simulink model "dcmg"  (R2020a)
settings: Solver=VariableStepAuto  StartTime=0.0  StopTime=Inf  FixedStep=50e-6  RelTol=1e-3
PostLoadFcn:
  | , if any(exist('dsrtsu_mdlpostloadfcn', 'file') ~= 0), dsrtsu_mdlpostloadfcn('Execute', bdroot); end,
InitFcn:
  | , if any(exist('rtifpga_mdlclblib', 'file') ~= 0), rtifpga_mdlclblib('Init', bdroot); end,
model workspace (MAT data in the model file):
  FPGA_dcmg_1_Register_1_1_1_write : Simulink.Signal (value not decoded)
  FPGA_dcmg_1_Register_2_1_1_write : Simulink.Signal (value not decoded)
  FPGA_dcmg_1_Register_3_1_1_write : Simulink.Signal (value not decoded)
  FPGA_dcmg_1_Register_4_1_1_write : Simulink.Signal (value not decoded)
  FPGA_dcmg_1_Register_5_1_1_write : Simulink.Signal (value not decoded)
values from neighbouring files (symbols this model uses):
  den = [1, zeros(1,499)]    [params.m]
  fixedgain_i = 10*1000/(3*100)    (= 33.3333333333)    [param.m]    (also in params.m)
  fixedgain_ibat = 10*1000/(3*100)    (= 33.3333333333)    [params.m]
  fixedgain_ipv = 10*1000/(3*100)    (= 33.3333333333)    [params.m]
  fixedgain_v = 10*22000/(3*100*2.5)    (= 293.333333333)    [params.m]
  fixedgain_vdc = 10*22000/(3*100*2.5)    (= 293.333333333)    [param.m]    (also in params.m = 586.666666667)
  fixedgain_vpv = 10*10000/(3*100*2.5)    (= 133.333333333)    [params.m]
  gain_iavsi = 1    [params.m]
  gain_ibat = 1    [params.m]
  gain_ibvsi = 1    [params.m]
  gain_icvsi = 1    [params.m]
  gain_ioavsi = 1    [params.m]
  gain_iobvsi = 1    [params.m]
  gain_ipv = 1    [params.m]
  gain_sinwave = 0.3    [params.m]
  gain_vavsi = 1    [params.m]
  gain_vbvsi = 1    [params.m]
  gain_vcvsi = 1    [params.m]
  gain_vdc = 1    [param.m]    (also in params.m)
  gain_vpv = 1    [params.m]
  N = 10    [param.m]    (also in params.m = 100)
  num = 1/500*ones(1,500)    [params.m]
  offset_iavsi = 0.2    [params.m]
  offset_ibat = 0    [params.m]
  offset_ibvsi = 0.2    [params.m]
  offset_icvsi = 0.2    [params.m]
  offset_ioavsi = 0    [params.m]
  offset_iobvsi = 0    [params.m]
  offset_ipv = 0    [params.m]
  offset_vavsi = 0    [params.m]
  offset_vbvsi = 0    [params.m]
  offset_vcvsi = 0    [params.m]
  offset_vdc = 1.5    [param.m]    (also in params.m = 0)
  offset_vpv = 0    [params.m]
  v_dc_ref = 40    [param.m]    (also in params.m = 24)
libraries: xbsIndex_r4 x258, rti1202lib_adc_class1 x10, rtiproclib x9, simulink x5, rti1202lib_adc_class2 x2, rtifpgainterfacelib x1
(part 7 of 7)

== system dcmg/fpga_dcmg/FPGA_XDATA_READ_BL1/phs_read_register/phs//rtlib_sim_model ==
  note: - The double to fixed-point conversion done by the XSG gateway behaves differently
      | than the conversion done by the RTLib C-code. Therefore the C-Code behaviour
      | is simulated via an s-function using the RTLib conversion technique including scaling and saturation.
  data_i1 : Inport
  S-Function : S-Function  FunctionName=DS1302_read_register  Parameters=mode;binaryPoint  SFunctionDeploymentMode=off  EnableBusSupport=off
  Zero-Order Hold : ZeroOrderHold  SampleTime=proc_sample_time
  data_o1 : Outport  VectorParamsAs1DForOutWhenUnconnected=off
  wires:
  Zero-Order Hold/1 -> S-Function/1
  S-Function/1 -> data_o1/1
  data_i1/1 -> Zero-Order Hold/1

== system dcmg/fpga_dcmg/FPGA_XDATA_READ_BL2/phs_read_register/com_fct_model ==
  note: - Register data is presented to the FPGA application without data adaptions.
      |
      | - Register group accesses are implicitly simulated by simulink: all FPGA
      | communication function interface blocks are simulated within one task
      | with a unique sample time --> in- and ouputs are sampled simultaneously
      | and therefore data consistency is guaranteed.
  data_i1 : Inport
  Data_New_Calc : Subsystem
  Zero-Order Hold : ZeroOrderHold  SampleTime=fpga_sample_time
  data_o1 : Outport  VectorParamsAs1DForOutWhenUnconnected=off
  data_new_o : Outport  Port=2  VectorParamsAs1DForOutWhenUnconnected=off
  wires:
  Zero-Order Hold/1 -> data_o1/1
  Data_New_Calc/1(Out1) -> data_new_o/1
  data_i1/1 -> Zero-Order Hold/1, Data_New_Calc/1(In1)

== system dcmg/fpga_dcmg/FPGA_XDATA_READ_BL2/phs_read_register/phs//rtlib_sim_model ==
  note: - The double to fixed-point conversion done by the XSG gateway behaves differently
      | than the conversion done by the RTLib C-code. Therefore the C-Code behaviour
      | is simulated via an s-function using the RTLib conversion technique including scaling and saturation.
  data_i1 : Inport
  S-Function : S-Function  FunctionName=DS1302_read_register  Parameters=mode;binaryPoint  SFunctionDeploymentMode=off  EnableBusSupport=off
  Zero-Order Hold : ZeroOrderHold  SampleTime=proc_sample_time
  data_o1 : Outport  VectorParamsAs1DForOutWhenUnconnected=off
  wires:
  Zero-Order Hold/1 -> S-Function/1
  S-Function/1 -> data_o1/1
  data_i1/1 -> Zero-Order Hold/1

== system dcmg/fpga_dcmg/FPGA_XDATA_READ_BL3/phs_read_register/com_fct_model ==
  note: - Register data is presented to the FPGA application without data adaptions.
      |
      | - Register group accesses are implicitly simulated by simulink: all FPGA
      | communication function interface blocks are simulated within one task
      | with a unique sample time --> in- and ouputs are sampled simultaneously
      | and therefore data consistency is guaranteed.
  data_i1 : Inport
  Data_New_Calc : Subsystem
  Zero-Order Hold : ZeroOrderHold  SampleTime=fpga_sample_time
  data_o1 : Outport  VectorParamsAs1DForOutWhenUnconnected=off
  data_new_o : Outport  Port=2  VectorParamsAs1DForOutWhenUnconnected=off
  wires:
  Zero-Order Hold/1 -> data_o1/1
  Data_New_Calc/1(Out1) -> data_new_o/1
  data_i1/1 -> Zero-Order Hold/1, Data_New_Calc/1(In1)

== system dcmg/fpga_dcmg/FPGA_XDATA_READ_BL3/phs_read_register/phs//rtlib_sim_model ==
  note: - The double to fixed-point conversion done by the XSG gateway behaves differently
      | than the conversion done by the RTLib C-code. Therefore the C-Code behaviour
      | is simulated via an s-function using the RTLib conversion technique including scaling and saturation.
  data_i1 : Inport
  S-Function : S-Function  FunctionName=DS1302_read_register  Parameters=mode;binaryPoint  SFunctionDeploymentMode=off  EnableBusSupport=off
  Zero-Order Hold : ZeroOrderHold  SampleTime=proc_sample_time
  data_o1 : Outport  VectorParamsAs1DForOutWhenUnconnected=off
  wires:
  Zero-Order Hold/1 -> S-Function/1
  S-Function/1 -> data_o1/1
  data_i1/1 -> Zero-Order Hold/1

== system dcmg/fpga_dcmg/FPGA_XDATA_READ_BL4/phs_read_register/com_fct_model ==
  note: - Register data is presented to the FPGA application without data adaptions.
      |
      | - Register group accesses are implicitly simulated by simulink: all FPGA
      | communication function interface blocks are simulated within one task
      | with a unique sample time --> in- and ouputs are sampled simultaneously
      | and therefore data consistency is guaranteed.
  data_i1 : Inport
  Data_New_Calc : Subsystem
  Zero-Order Hold : ZeroOrderHold  SampleTime=fpga_sample_time
  data_o1 : Outport  VectorParamsAs1DForOutWhenUnconnected=off
  data_new_o : Outport  Port=2  VectorParamsAs1DForOutWhenUnconnected=off
  wires:
  Zero-Order Hold/1 -> data_o1/1
  Data_New_Calc/1(Out1) -> data_new_o/1
  data_i1/1 -> Zero-Order Hold/1, Data_New_Calc/1(In1)

== system dcmg/fpga_dcmg/FPGA_XDATA_READ_BL4/phs_read_register/phs//rtlib_sim_model ==
  note: - The double to fixed-point conversion done by the XSG gateway behaves differently
      | than the conversion done by the RTLib C-code. Therefore the C-Code behaviour
      | is simulated via an s-function using the RTLib conversion technique including scaling and saturation.
  data_i1 : Inport
  S-Function : S-Function  FunctionName=DS1302_read_register  Parameters=mode;binaryPoint  SFunctionDeploymentMode=off  EnableBusSupport=off
  Zero-Order Hold : ZeroOrderHold  SampleTime=proc_sample_time
  data_o1 : Outport  VectorParamsAs1DForOutWhenUnconnected=off
  wires:
  Zero-Order Hold/1 -> S-Function/1
  S-Function/1 -> data_o1/1
  data_i1/1 -> Zero-Order Hold/1

== system dcmg/fpga_dcmg/FPGA_XDATA_READ_BL5/phs_read_register/com_fct_model ==
  note: - Register data is presented to the FPGA application without data adaptions.
      |
      | - Register group accesses are implicitly simulated by simulink: all FPGA
      | communication function interface blocks are simulated within one task
      | with a unique sample time --> in- and ouputs are sampled simultaneously
      | and therefore data consistency is guaranteed.
  data_i1 : Inport
  Data_New_Calc : Subsystem
  Zero-Order Hold : ZeroOrderHold  SampleTime=fpga_sample_time
  data_o1 : Outport  VectorParamsAs1DForOutWhenUnconnected=off
  data_new_o : Outport  Port=2  VectorParamsAs1DForOutWhenUnconnected=off
  wires:
  Zero-Order Hold/1 -> data_o1/1
  Data_New_Calc/1(Out1) -> data_new_o/1
  data_i1/1 -> Zero-Order Hold/1, Data_New_Calc/1(In1)

== system dcmg/fpga_dcmg/FPGA_XDATA_READ_BL5/phs_read_register/phs//rtlib_sim_model ==
  note: - The double to fixed-point conversion done by the XSG gateway behaves differently
      | than the conversion done by the RTLib C-code. Therefore the C-Code behaviour
      | is simulated via an s-function using the RTLib conversion technique including scaling and saturation.
  data_i1 : Inport
  S-Function : S-Function  FunctionName=DS1302_read_register  Parameters=mode;binaryPoint  SFunctionDeploymentMode=off  EnableBusSupport=off
  Zero-Order Hold : ZeroOrderHold  SampleTime=proc_sample_time
  data_o1 : Outport  VectorParamsAs1DForOutWhenUnconnected=off
  wires:
  Zero-Order Hold/1 -> S-Function/1
  S-Function/1 -> data_o1/1
  data_i1/1 -> Zero-Order Hold/1

== system dcmg/RTI Data/RTI Data Store/RTI Data Store/RTI Data Store/RTI Data Store ==

== system dcmg/fpga_dcmg/FPGA_INT_BL1/phs_interrupt/phs//rtlib_sim_model/Triggered Subsystem ==
  Trigger : TriggerPort  VariantControl=(inherit)
  Function-Call Generator : simulink/Ports & Subsystems/Function-Call Generator  sample_time=-1  numberOfIterations=1
  Out1 : Outport  VectorParamsAs1DForOutWhenUnconnected=off
  wires:
  Function-Call Generator/1 -> Out1/1

== system dcmg/fpga_dcmg/FPGA_INT_BL2/phs_interrupt/phs//rtlib_sim_model/Triggered Subsystem ==
  Trigger : TriggerPort  VariantControl=(inherit)
  Function-Call Generator : simulink/Ports & Subsystems/Function-Call Generator  sample_time=-1  numberOfIterations=1
  Out1 : Outport  VectorParamsAs1DForOutWhenUnconnected=off
  wires:
  Function-Call Generator/1 -> Out1/1

== system dcmg/fpga_dcmg/FPGA_INT_BL3/phs_interrupt/phs//rtlib_sim_model/Triggered Subsystem ==
  Trigger : TriggerPort  VariantControl=(inherit)
  Function-Call Generator : simulink/Ports & Subsystems/Function-Call Generator  sample_time=-1  numberOfIterations=1
  Out1 : Outport  VectorParamsAs1DForOutWhenUnconnected=off
  wires:
  Function-Call Generator/1 -> Out1/1

== system dcmg/fpga_dcmg/FPGA_XDATA_READ_BL1/phs_read_register/com_fct_model/Data_New_Calc ==
  note: The new data flag is presented whenever the input data port is sampled.
      | The flag is set to 1 for one FPGA simulation step and reset to 0 for the
      | remaining FPGA simulation steps contained within one processor simulation step.
  In1 : Inport
  Add : Sum
  Constant : Constant  Value=fpga_sample_time  SampleTime=fpga_sample_time
  Constant1 : Constant  Value=0
  Divide : Product  Inputs=*/
  Divide1 : Product  Inputs=*/
  Math Function : Math  Operator=mod  SignedPower=on  SaturateOnIntegerOverflow=on
  Relational Operator : RelationalOperator  Operator===  OutDataTypeStr=boolean  RndMeth=Nearest
  Unit Delay1 : UnitDelay  InitialCondition=-1  SampleTime=-1  HasFrameUpgradeWarning=on
  Weighted Sample Time1 : SampleTimeMath  TsampMathOp=Ts Only
  Out1 : Outport  VectorParamsAs1DForOutWhenUnconnected=off
  wires:
  Constant/1 -> Divide1/2, Divide1/1, Divide/2
  Weighted Sample Time1/1 -> Divide/1
  Math Function/1 -> Relational Operator/1
  Relational Operator/1 -> Out1/1
  In1/1 -> Weighted Sample Time1/1
  Divide1/1 -> Add/1
  Unit Delay1/1 -> Add/2
  Add/1 -> Unit Delay1/1, Math Function/1
  Constant1/1 -> Relational Operator/2
  Divide/1 -> Math Function/2

== system dcmg/fpga_dcmg/FPGA_XDATA_READ_BL2/phs_read_register/com_fct_model/Data_New_Calc ==
  note: The new data flag is presented whenever the input data port is sampled.
      | The flag is set to 1 for one FPGA simulation step and reset to 0 for the
      | remaining FPGA simulation steps contained within one processor simulation step.
  In1 : Inport
  Add : Sum
  Constant : Constant  Value=fpga_sample_time  SampleTime=fpga_sample_time
  Constant1 : Constant  Value=0
  Divide : Product  Inputs=*/
  Divide1 : Product  Inputs=*/
  Math Function : Math  Operator=mod  SignedPower=on  SaturateOnIntegerOverflow=on
  Relational Operator : RelationalOperator  Operator===  OutDataTypeStr=boolean  RndMeth=Nearest
  Unit Delay1 : UnitDelay  InitialCondition=-1  SampleTime=-1  HasFrameUpgradeWarning=on
  Weighted Sample Time1 : SampleTimeMath  TsampMathOp=Ts Only
  Out1 : Outport  VectorParamsAs1DForOutWhenUnconnected=off
  wires:
  Constant/1 -> Divide1/2, Divide1/1, Divide/2
  Weighted Sample Time1/1 -> Divide/1
  Math Function/1 -> Relational Operator/1
  Relational Operator/1 -> Out1/1
  In1/1 -> Weighted Sample Time1/1
  Divide1/1 -> Add/1
  Unit Delay1/1 -> Add/2
  Add/1 -> Unit Delay1/1, Math Function/1
  Constant1/1 -> Relational Operator/2
  Divide/1 -> Math Function/2

== system dcmg/fpga_dcmg/FPGA_XDATA_READ_BL3/phs_read_register/com_fct_model/Data_New_Calc ==
  note: The new data flag is presented whenever the input data port is sampled.
      | The flag is set to 1 for one FPGA simulation step and reset to 0 for the
      | remaining FPGA simulation steps contained within one processor simulation step.
  In1 : Inport
  Add : Sum
  Constant : Constant  Value=fpga_sample_time  SampleTime=fpga_sample_time
  Constant1 : Constant  Value=0
  Divide : Product  Inputs=*/
  Divide1 : Product  Inputs=*/
  Math Function : Math  Operator=mod  SignedPower=on  SaturateOnIntegerOverflow=on
  Relational Operator : RelationalOperator  Operator===  OutDataTypeStr=boolean  RndMeth=Nearest
  Unit Delay1 : UnitDelay  InitialCondition=-1  SampleTime=-1  HasFrameUpgradeWarning=on
  Weighted Sample Time1 : SampleTimeMath  TsampMathOp=Ts Only
  Out1 : Outport  VectorParamsAs1DForOutWhenUnconnected=off
  wires:
  Constant/1 -> Divide1/2, Divide1/1, Divide/2
  Weighted Sample Time1/1 -> Divide/1
  Math Function/1 -> Relational Operator/1
  Relational Operator/1 -> Out1/1
  In1/1 -> Weighted Sample Time1/1
  Divide1/1 -> Add/1
  Unit Delay1/1 -> Add/2
  Add/1 -> Unit Delay1/1, Math Function/1
  Constant1/1 -> Relational Operator/2
  Divide/1 -> Math Function/2

== system dcmg/fpga_dcmg/FPGA_XDATA_READ_BL4/phs_read_register/com_fct_model/Data_New_Calc ==
  note: The new data flag is presented whenever the input data port is sampled.
      | The flag is set to 1 for one FPGA simulation step and reset to 0 for the
      | remaining FPGA simulation steps contained within one processor simulation step.
  In1 : Inport
  Add : Sum
  Constant : Constant  Value=fpga_sample_time  SampleTime=fpga_sample_time
  Constant1 : Constant  Value=0
  Divide : Product  Inputs=*/
  Divide1 : Product  Inputs=*/
  Math Function : Math  Operator=mod  SignedPower=on  SaturateOnIntegerOverflow=on
  Relational Operator : RelationalOperator  Operator===  OutDataTypeStr=boolean  RndMeth=Nearest
  Unit Delay1 : UnitDelay  InitialCondition=-1  SampleTime=-1  HasFrameUpgradeWarning=on
  Weighted Sample Time1 : SampleTimeMath  TsampMathOp=Ts Only
  Out1 : Outport  VectorParamsAs1DForOutWhenUnconnected=off
  wires:
  Constant/1 -> Divide1/2, Divide1/1, Divide/2
  Weighted Sample Time1/1 -> Divide/1
  Math Function/1 -> Relational Operator/1
  Relational Operator/1 -> Out1/1
  In1/1 -> Weighted Sample Time1/1
  Divide1/1 -> Add/1
  Unit Delay1/1 -> Add/2
  Add/1 -> Unit Delay1/1, Math Function/1
  Constant1/1 -> Relational Operator/2
  Divide/1 -> Math Function/2

== system dcmg/fpga_dcmg/FPGA_XDATA_READ_BL5/phs_read_register/com_fct_model/Data_New_Calc ==
  note: The new data flag is presented whenever the input data port is sampled.
      | The flag is set to 1 for one FPGA simulation step and reset to 0 for the
      | remaining FPGA simulation steps contained within one processor simulation step.
  In1 : Inport
  Add : Sum
  Constant : Constant  Value=fpga_sample_time  SampleTime=fpga_sample_time
  Constant1 : Constant  Value=0
  Divide : Product  Inputs=*/
  Divide1 : Product  Inputs=*/
  Math Function : Math  Operator=mod  SignedPower=on  SaturateOnIntegerOverflow=on
  Relational Operator : RelationalOperator  Operator===  OutDataTypeStr=boolean  RndMeth=Nearest
  Unit Delay1 : UnitDelay  InitialCondition=-1  SampleTime=-1  HasFrameUpgradeWarning=on
  Weighted Sample Time1 : SampleTimeMath  TsampMathOp=Ts Only
  Out1 : Outport  VectorParamsAs1DForOutWhenUnconnected=off
  wires:
  Constant/1 -> Divide1/2, Divide1/1, Divide/2
  Weighted Sample Time1/1 -> Divide/1
  Math Function/1 -> Relational Operator/1
  Relational Operator/1 -> Out1/1
  In1/1 -> Weighted Sample Time1/1
  Divide1/1 -> Add/1
  Unit Delay1/1 -> Add/2
  Add/1 -> Unit Delay1/1, Math Function/1
  Constant1/1 -> Relational Operator/2
  Divide/1 -> Math Function/2

== matlab function dcmg/MPPT_system/MATLAB Function ==
  data: v_pv input; v_PandO output; i input; v_dc input; d output; P output
function [v_PandO, d, P] = MPPT(v_pv,i, v_dc)
persistent P_ant v_ref v_ant v_dc_ant

if isempty(P_ant)
    P_ant = 0;
    v_ref = 28;
    v_ant = 28;
end


P = v_pv*i;

v_dc_ant = v_dc;
delta = P-P_ant;

if (abs(delta) < 0.001)
elseif delta > 0
        if v_pv>v_ant
            v_ref = v_ref+.1;
        else
            v_ref = v_ref-.1;
        end
else
        if v_pv>v_ant
            v_ref = v_ref-.1;
        else
            v_ref = v_ref+.1;
        end
end
if v_ref>35.9
    v_ref = 35.9;
end
if v_ref<0
    v_ref = 0;
end
P_ant = P;
v_ant = v_pv;

v_PandO = v_ref;


g = v_dc_ant/v_ref;
d = 100*(1-(1/g));
if d<1
    d = 1;
elseif d>99
    d=99;
end
